simulink model "ai_optimal_path_v1_3"  (R2019a)
settings: Solver=FixedStepDiscrete  StartTime=0.0  StopTime=inf  FixedStep=0.2  RelTol=1e-3  EnableMultiTasking=on
undefined symbols (not defined in the file): Data, Data_SL_Info
libraries: robotlib x15
(part 2 of 2)

== matlab function ai_optimal_path_v1_3/MATLAB Function8 ==
  data: octomap_center input size=[650000 3]; Obstacle output size=[100 100 25]; pos_init input
function Obstacle = gen_3d_array(octomap_center,pos_init)

mapsize = [100 100 25];

Obstacle = int8(zeros(mapsize(1),mapsize(2),mapsize(3)));
grid_size = 0.2;
start_point = [pos_init(1) pos_init(2) pos_init(3)];

% align1 = int16(octomap_center/(grid_size)+0.5);
align1 = int16(octomap_center/(grid_size));
align2 = unique(align1,'rows');
align3 = [align2(:,1)+start_point(1) align2(:,2)+start_point(2) align2(:,3)+start_point(3)];

for i = 1:numel(align3)/3
    
    index_temp = align3(i,:);
    
    index_check = index_temp<3;
    if sum(index_check)>=1
        index_temp(index_check) = 3;
    end
    
    if index_temp(1) > mapsize(1)-2
        index_temp(1) = mapsize(1)-2;
    end
    if index_temp(2) > mapsize(2)-2
        index_temp(2) = mapsize(2)-2;
    end
    if index_temp(3) > mapsize(3)-2
        index_temp(3) = mapsize(3)-2;
    end
    

    index_x = index_temp(1)-2:index_temp(1)+2;
    index_y = index_temp(2)-1:index_temp(2)+1;
    index_z = index_temp(3)-1:index_temp(3)+1;
%------------------------------------------------------------------------
%-----------------------------  scattering  -----------------------------
%------------------------------------------------------------------------
    Obstacle(index_x,index_temp(2)+1,index_temp(3)+1) = 1;
    Obstacle(index_x,index_temp(2)+1,index_temp(3)) = 1;
    Obstacle(index_x,index_temp(2)+1,index_temp(3)-1) = 1;
    Obstacle(index_x,index_temp(2),index_temp(3)+1) = 1;
    Obstacle(index_x,index_temp(2),index_temp(3)) = 1;
    Obstacle(index_x,index_temp(2),index_temp(3)-1) = 1;
    Obstacle(index_x,index_temp(2)-1,index_temp(3)+1) = 1;
    Obstacle(index_x,index_temp(2)-1,index_temp(3)) = 1;
    Obstacle(index_x,index_temp(2)-1,index_temp(3)-1) = 1;
    
    Obstacle(index_temp(1)+1,index_temp(2)+2,index_z) = 1;
    Obstacle(index_temp(1)+1,index_temp(2)-2,index_z) = 1;
    Obstacle(index_temp(1),index_temp(2)+2,index_z) = 1;
    Obstacle(index_temp(1),index_temp(2)-2,index_z) = 1;
    Obstacle(index_temp(1)-1,index_temp(2)+2,index_z) = 1;
    Obstacle(index_temp(1)-1,index_temp(2)-2,index_z) = 1;
    
    
    
    Obstacle(index_temp(1),index_y,index_temp(3)+2) = 1;
    Obstacle(index_temp(1),index_y,index_temp(3)-2) = 1;
    Obstacle(index_temp(1)+1,index_y,index_temp(3)+2) = 1;
    Obstacle(index_temp(1)+1,index_y,index_temp(3)-2) = 1;
    Obstacle(index_temp(1)-1,index_y,index_temp(3)+2) = 1;
    Obstacle(index_temp(1)-1,index_y,index_temp(3)-2) = 1;  %  Z FLAT Vehicle
    
    
    

%------------------------------------------------------------------------
%----------------------------  scattering 2  ----------------------------
%------------------------------------------------------------------------
    Obstacle(index_temp(1)+2,index_temp(2)+2,index_z) = 1;
    Obstacle(index_temp(1)+2,index_temp(2)+1,index_z) = 1;
    Obstacle(index_temp(1)+2,index_temp(2),index_z) = 1;
    Obstacle(index_temp(1)+2,index_temp(2)-1,index_z) = 1;
    Obstacle(index_temp(1)+2,index_temp(2)-2,index_z) = 1;
    
    Obstacle(index_temp(1)+1,index_temp(2)+2,index_z) = 1;
    Obstacle(index_temp(1)+1,index_temp(2)+1,index_z) = 1;
    Obstacle(index_temp(1)+1,index_temp(2),index_z) = 1;
    Obstacle(index_temp(1)+1,index_temp(2)-1,index_z) = 1;
    Obstacle(index_temp(1)+1,index_temp(2)-2,index_z) = 1;
    
    Obstacle(index_temp(1),index_temp(2)+2,index_z) = 1;
    Obstacle(index_temp(1),index_temp(2)+1,index_z) = 1;
    Obstacle(index_temp(1),index_temp(2),index_z) = 1;
    Obstacle(index_temp(1),index_temp(2)-1,index_z) = 1;
    Obstacle(index_temp(1),index_temp(2)-2,index_z) = 1;
    
    Obstacle(index_temp(1)-1,index_temp(2)+2,index_z) = 1;
    Obstacle(index_temp(1)-1,index_temp(2)+1,index_z) = 1;
    Obstacle(index_temp(1)-1,index_temp(2),index_z) = 1;
    Obstacle(index_temp(1)-1,index_temp(2)-1,index_z) = 1;
    Obstacle(index_temp(1)-1,index_temp(2)-2,index_z) = 1;
    
    Obstacle(index_temp(1)-2,index_temp(2)+2,index_z) = 1;
    Obstacle(index_temp(1)-2,index_temp(2)+1,index_z) = 1;
    Obstacle(index_temp(1)-2,index_temp(2),index_z) = 1;
    Obstacle(index_temp(1)-2,index_temp(2)-1,index_z) = 1;
    Obstacle(index_temp(1)-2,index_temp(2)-2,index_z) = 1;
    
end

Obstacle(1:3,:,:)=1;
Obstacle(mapsize(1)-2:mapsize(1),:,:) = 1;
Obstacle(:,1:3,:) = 1;
Obstacle(:,mapsize(2)-2:mapsize(2),:) = 1;
Obstacle(:,:,1:3) = 1;
% Obstacle(:,:,mapsize(3)-10:mapsize(3)) = 1; % 고도제한 2m 
Obstacle(:,:,mapsize(3)-8:mapsize(3)) = 1; % 고도제한 2.4m 

end

== matlab function ai_optimal_path_v1_3/MATLAB Function9 ==
  data: data input size=[128 1]; test output size=[1 128]; SL output
function [test,SL]   = func(data)

% test = single(nan(1,128));

test = data';
% for i = 1:length(data)
%     test(i) = single(data(i));
% end

SL = uint32(length(data));


end
